simulink model "EKF1"  (R2017a)
settings: Solver=FixedStepAuto  StartTime=0.0  StopTime=50.0  FixedStep=0.1  RelTol=1e-3
libraries: simulink x2
settings Model: Creator=Soutrik  LastModifiedBy=Soutrik

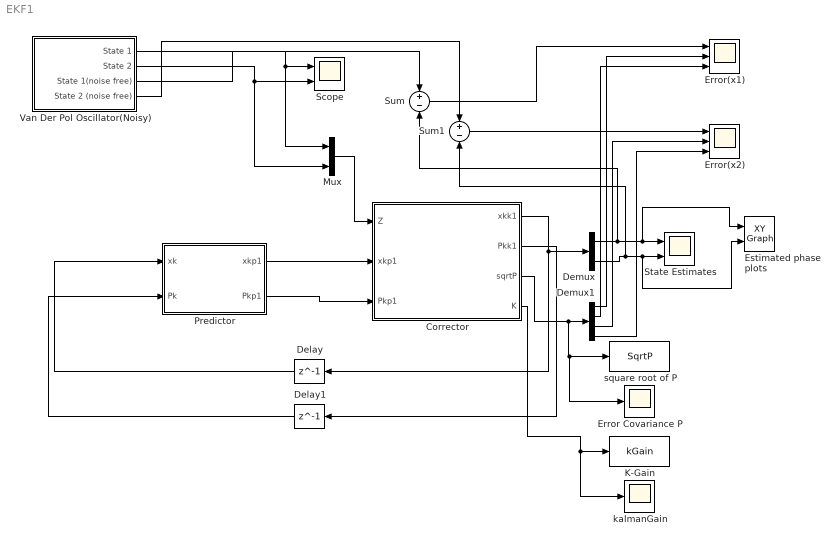
== system EKF1 ==
  Corrector : MATLAB Function  TreatAsAtomicUnit=on
  Delay : Delay  DelayLength=1  InitialCondition=[-0.5;0.5]
  Delay1 : Delay  DelayLength=1  InitialCondition=eye(2)
  Demux : Demux  Outputs=2
  Demux1 : Demux
  Error Covariance P : Scope
  Error(x1) : Scope  NumInputPorts=3
  Error(x2) : Scope  NumInputPorts=3
  Estimated phase plots : simulink/Sinks/XY Graph  xmin=-3  xmax=3  ymin=-3  ymax=3  st=-1
  K-Gain : ToWorkspace  VariableName=kGain  SampleTime=-1
  Mux : Mux  Inputs=2
  Predictor : MATLAB Function  TreatAsAtomicUnit=on
  Scope : Scope  NumInputPorts=2
  State Estimates : Scope  NumInputPorts=2
  Sum : Sum  Inputs=+-
  Sum1 : Sum  Inputs=+-
  Van Der Pol Oscillator(Noisy) : Subsystem
  kalmanGain : Scope
  square root of P : ToWorkspace  VariableName=SqrtP  SampleTime=-1
  wires:
  Van Der Pol Oscillator(Noisy)/1(State 1) -> Mux/1, Scope/1
  Van Der Pol Oscillator(Noisy)/2(State 2) -> Mux/2, Scope/2
  Mux/1 -> Corrector/1(Z)
  Corrector/1(xkk1) -> Demux/1, Delay/1
  Delay/1 -> Predictor/1(xk)
  Corrector/2(Pkk1) -> Delay1/1
  Delay1/1 -> Predictor/2(Pk)
  Predictor/1(xkp1) -> Corrector/2(xkp1)
  Predictor/2(Pkp1) -> Corrector/3(Pkp1)
  Demux/1 -> Sum/2, State Estimates/1, Estimated phase plots/1
  Demux/2 -> Sum1/2, State Estimates/2, Estimated phase plots/2
  Sum/1 -> Error(x1)/1
  Van Der Pol Oscillator(Noisy)/3(State 1(noise free)) -> Sum/1
  Van Der Pol Oscillator(Noisy)/4(State 2 (noise free)) -> Sum1/1
  Corrector/3(sqrtP) -> Error Covariance P/1, square root of P/1, Demux1/1
  Sum1/1 -> Error(x2)/1
  Corrector/4(K) -> kalmanGain/1, K-Gain/1
  Demux1/1 -> Error(x1)/2
  Demux1/2 -> Error(x1)/3
  Demux1/3 -> Error(x2)/2
  Demux1/4 -> Error(x2)/3

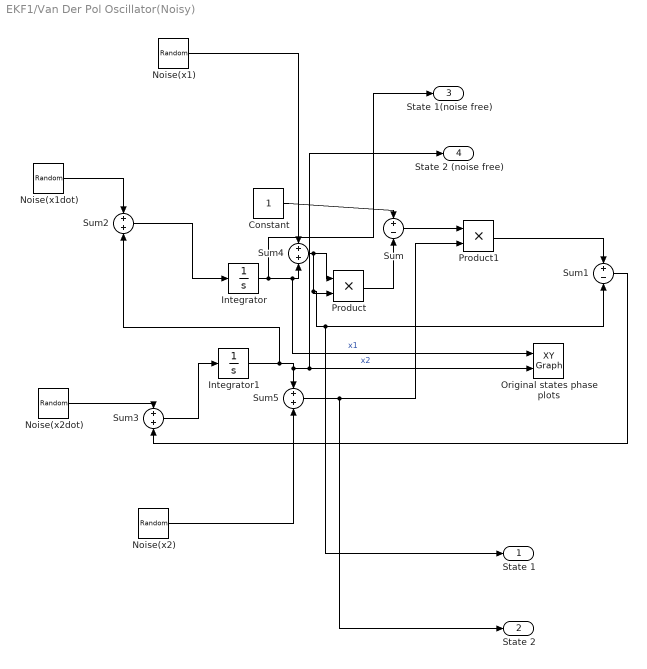
== system EKF1/Van Der Pol Oscillator(Noisy) ==
  Constant : Constant
  Integrator : Integrator  InitialCondition=0.1
  Integrator1 : Integrator  InitialCondition=0.1
  Noise(x1) : RandomNumber  Variance=0.015  Seed=73  SampleTime=0.1
  Noise(x1dot) : RandomNumber  Variance=0.2  Seed=43  SampleTime=0.1
  Noise(x2) : RandomNumber  Variance=0.025  Seed=87  SampleTime=0.1
  Noise(x2dot) : RandomNumber  Variance=0.1  Seed=57  SampleTime=0.1
  Original states phase plots : simulink/Sinks/XY Graph  xmin=-3  xmax=3  ymin=-3  ymax=3  st=0.1
  Product : Product
  Product1 : Product
  Sum : Sum  Inputs=+-
  Sum1 : Sum  Inputs=+-
  Sum{2..5} (4 alike) : Sum  Inputs=2
  State 1 : Outport
  State 2 : Outport  Port=2
  State 1(noise free) : Outport  Port=3
  State 2 (noise free) : Outport  Port=4
  wires:
  Sum3/1 -> Integrator1/1
  Sum2/1 -> Integrator/1
  Constant/1 -> Sum/1
  Sum/1 -> Product1/1
  Product/1 -> Sum/2
  Noise(x2)/1 -> Sum5/2
  Noise(x1dot)/1 -> Sum2/1
  Sum4/1 -> State 1/1, Sum1/2, Product/2, Product/1
  Noise(x2dot)/1 -> Sum3/1
  Noise(x1)/1 -> Sum4/1
  Sum1/1 -> Sum3/2
  Product1/1 -> Sum1/1
  Integrator/1 -> State 1(noise free)/1, Original states phase plots/1, Sum4/2  "x1"
  Integrator1/1 -> Sum2/2, Original states phase plots/2, State 2 (noise free)/1, Sum5/1  "x2"
  Sum5/1 -> State 2/1, Product1/2

== matlab function EKF1/Corrector ==
  data: Z input; xkk1 output; xkp1 input; Pkp1 input; Pkk1 output; sqrtP output; K output
function [xkk1, Pkk1,sqrtP,K] = corrector(Z,xkp1,Pkp1)

xkk1=zeros(2,1);
Pkk1=zeros(2);
sqrtP=zeros(4,1);


R=diag([0.4, 0.2]);

H=eye(2);
dh=eye(2);

K=Pkp1*dh'*inv(dh*Pkp1*(dh)'+R);
Pkk1=Pkp1- K*(dh*Pkp1*(dh)'+R)*K';
xkk1=xkp1+K*(Z-H*xkp1);

P22=Pkk1(2,2)
sqrtP(4,1)=sqrt(P22);
sqrtP(3,1)=-sqrt(P22);
P11=Pkk1(1,1)
sqrtP(2,1)=sqrt(P11);
sqrtP(1,1)=-sqrt(P11);

end

== matlab function EKF1/Predictor ==
  data: xk input; xkp1 output; Pk input; Pkp1 output
function [xkp1, Pkp1] = predictor(xk, Pk)

xkp1=zeros(2,1);
Pkp1=zeros(2);

x1=xk(1);
x2=xk(2);
a =[0 1; -2*x1*x2-1 1-x1*x1];

Q = diag([2 2]);
%Pk=eye(2);
T=0.1;
Ad=expm(a*T);

F=[-a Q;zeros(2,2) a'];
G=expm(F*T);
GLr=G(3:4,3:4);
Gur=G(1:2,3:4);
Qd=GLr'*Gur;

xkp1=Ad*xk;
Pkp1=Ad*Pk*Ad'+Qd;

end
